simulink model "bee_scratch"  (Simulink 7.0)
settings: Solver=ode45  StartTime=0.0  StopTime=600  RelTol=1e-3
libraries: xbsIndex_r4 x52, xps_library x7, casper_library x2
settings Model: Creator=Laura  LastModifiedBy=Laura

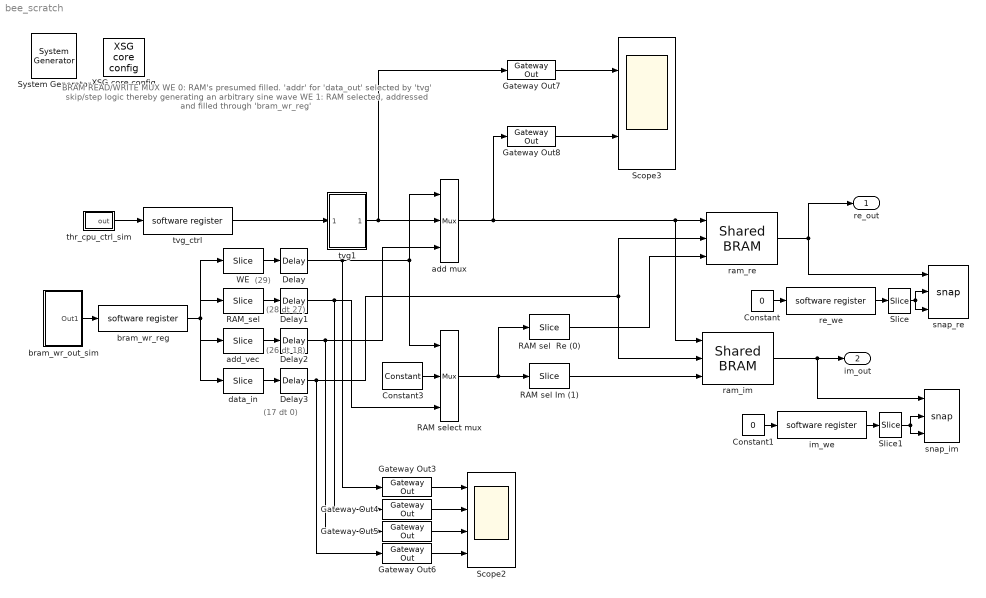
== system bee_scratch ==
  note: BRAM READ/WRITE MUX
      | WE 0: RAM's presumed filled.
      | 'addr' for 'data_out' selected
      | by 'tvg' skip/step logic thereby
      | generating an arbitrary sine wave
      | WE 1: RAM selected, addressed
      | and filled through
      | 'bram_wr_reg'
  note: (29)
  note: (28 dt 27)
  note: (17 dt 0)
  note: (26 dt 18)
  " System Generator" : xbsIndex_r4/ System Generator  Tag=genX  SystemSampleTime=-1  xilinxfamily=virtex2p  part=xc2vp70  speed=-7  package=ff1704  synthesis_tool=XST  clock_wrapper=Clock Enables  directory=./bee_scratch/sysgen  testbench=off  simulink_period=1  sysclk_period=5  dcm_input_clock_period=100  incr_netlist=off  trim_vbits=Everywhere in SubSystem  dbl_ovrd=According to Block Masks  core_generation=According to Block Masks  run_coregen=off  deprecated_control=off  eval_field=0  block_type=sysgen
      settings: block_version=10.1.2
  Constant : Constant  Value=0  OutDataType=sfix(16)  OutScaling=2^0
  Constant1 : Constant  Value=0  OutDataType=sfix(16)  OutScaling=2^0
  Constant3 : xbsIndex_r4/Constant  arith_type=Unsigned  const=0  n_bits=4  bin_pt=0  explicit_period=on  period=1  equ=P=C  opselect=C  inp2=PCIN>>17  opr=+  inp1=P  carry=CIN  dbl_ovrd=off  block_type=constant
      settings: block_version=10.1.2
  Delay{,1..3} (4 alike) : xbsIndex_r4/Delay  en=off  latency=1  dbl_ovrd=off  reg_retiming=off  block_type=delay
      settings: xl_area=[0, 0, 0, 0, 0, 0, 0]  block_version=10.1.2
  Gateway Out{3..8} (6 alike) : xbsIndex_r4/Gateway Out  hdl_port=on  timing_constraint=None  locs_specified=off  LOCs={}  block_type=gatewayout
      settings: infoedit="Gateway out block.  Converts Xilinx fixed point inputs into ouputs of type Simulink integer, double, or fixed point.<P><P>Hardware notes:  In hardware these blocks become top level output ports or are discarded, depending on how they are configured."  xl_area=[0, 0, 0, 0, 0, 0, 0]  block_version=10.1.2
  RAM sel  Re (0) : xbsIndex_r4/Slice  nbits=1  boolean_output=on  mode=Lower Bit Location + Width  bit1=0  base1=MSB of Input  bit0=0  base0=LSB of Input  dbl_ovrd=off  block_type=slice
      settings: infoedit="Extracts a given range of bits from each input sample and presents it at the output.  The output type is ordinarily unsigned with binary point at zero, but can be Boolean when the slice is one bit wide.<P><P>Hardware notes: In hardware this block costs nothing."  block_version=10.1.2
  RAM sel Im (1) : xbsIndex_r4/Slice  nbits=1  boolean_output=on  mode=Lower Bit Location + Width  bit1=0  base1=MSB of Input  bit0=1  base0=LSB of Input  dbl_ovrd=off  block_type=slice
      settings: infoedit="Extracts a given range of bits from each input sample and presents it at the output.  The output type is ordinarily unsigned with binary point at zero, but can be Boolean when the slice is one bit wide.<P><P>Hardware notes: In hardware this block costs nothing."  block_version=10.1.2
  RAM select mux : xbsIndex_r4/Mux  inputs=2  en=off  latency=0  precision=Full  arith_type="Signed  (2's comp)"  n_bits=8  bin_pt=2  quantization=Truncate  overflow=Wrap  dbl_ovrd=off  block_type=mux
      settings: xl_area=[0, 0, 0, 0, 0, 0, 0]  block_version=10.1.2
  RAM_sel : xbsIndex_r4/Slice  nbits=2  boolean_output=off  mode=Lower Bit Location + Width  bit1=10  base1=MSB of Input  bit0=27  base0=LSB of Input  dbl_ovrd=off  block_type=slice
      settings: infoedit="Extracts a given range of bits from each input sample and presents it at the output.  The output type is ordinarily unsigned with binary point at zero, but can be Boolean when the slice is one bit wide.<P><P>Hardware notes: In hardware this block costs nothing."  block_version=10.1.2
  Scope2 : Scope  NumInputPorts=4
      settings: YMin=-5~-5~-5~-5  YMax=5~5~5~5
  Scope3 : Scope  NumInputPorts=2
      settings: YMin=-5~-5  YMax=5~5  SaveName=ScopeData3
  Slice : xbsIndex_r4/Slice  nbits=1  boolean_output=on  mode=Lower Bit Location + Width  bit1=0  base1=MSB of Input  bit0=0  base0=LSB of Input  dbl_ovrd=off  block_type=slice
      settings: infoedit="Extracts a given range of bits from each input sample and presents it at the output.  The output type is ordinarily unsigned with binary point at zero, but can be Boolean when the slice is one bit wide.<P><P>Hardware notes: In hardware this block costs nothing."  block_version=10.1.2
  Slice1 : xbsIndex_r4/Slice  nbits=1  boolean_output=on  mode=Lower Bit Location + Width  bit1=0  base1=MSB of Input  bit0=0  base0=LSB of Input  dbl_ovrd=off  block_type=slice
      settings: infoedit="Extracts a given range of bits from each input sample and presents it at the output.  The output type is ordinarily unsigned with binary point at zero, but can be Boolean when the slice is one bit wide.<P><P>Hardware notes: In hardware this block costs nothing."  block_version=10.1.2
  WE : xbsIndex_r4/Slice  nbits=1  boolean_output=off  mode=Lower Bit Location + Width  bit1=10  base1=MSB of Input  bit0=29  base0=LSB of Input  dbl_ovrd=off  block_type=slice
      settings: infoedit="Extracts a given range of bits from each input sample and presents it at the output.  The output type is ordinarily unsigned with binary point at zero, but can be Boolean when the slice is one bit wide.<P><P>Hardware notes: In hardware this block costs nothing."  block_version=10.1.2
  XSG core config : xps_library/XSG core config  Tag=xps:xsg  SystemSampleTime=-1  hw_sys=BEE2_usr  ibob_linux=off  clk_src=usr_clk2x  gpio_clk_io_group=iBOB:sma  gpio_clk_bit_index=0  clk_rate=200  sample_period=1  synthesis_tool=XST  mpc_type=powerpc405
  add mux : xbsIndex_r4/Mux  inputs=2  en=off  latency=0  precision=Full  arith_type="Signed  (2's comp)"  n_bits=8  bin_pt=2  quantization=Truncate  overflow=Wrap  dbl_ovrd=off  block_type=mux
      settings: xl_area=[0, 0, 0, 0, 0, 0, 0]  block_version=10.1.2
  add_vec : xbsIndex_r4/Slice  nbits=9  boolean_output=off  mode=Lower Bit Location + Width  bit1=0  base1=MSB of Input  bit0=18  base0=LSB of Input  dbl_ovrd=off  block_type=slice
      settings: infoedit="Extracts a given range of bits from each input sample and presents it at the output.  The output type is ordinarily unsigned with binary point at zero, but can be Boolean when the slice is one bit wide.<P><P>Hardware notes: In hardware this block costs nothing."  block_version=10.1.2
  bram_wr_out_sim : Subsystem  mask{we_enable=0, ram_sel=3, add_vec=512, data_in=32}
      mask prompts: we_enable "Write enable"; ram_sel "RAM selector (1 = Re; 2 = Im; 3 = both)"; add_vec "RAM address"; data_in "Data in"
  bram_wr_reg : xps_library/software register  Tag=xps:sw_reg  SystemSampleTime=-1  io_dir=From Processor  arith_type=Unsigned  bitwidth=32  bin_pt=0  sample_period=1  gw_name=bee_scratch_bram_wr_reg_user_data_out
      link override bee_scratch_bram_wr_reg_user_data_out: arith_type=Unsigned  n_bits=32  bin_pt=0  period=1
      link override bee_scratch_data_in_mux_tvg_in_bram_wr_reg_user_data_out: arith_type=Unsigned  n_bits=32  bin_pt=0  period=1
      link override bee_scratch_tvg_bram_wr_reg_user_data_out: arith_type=Unsigned  n_bits=32  bin_pt=0  period=1
      link override bee_scratch_tvg_in_bram_wr_reg_user_data_out: arith_type=Unsigned  n_bits=32  bin_pt=0  period=1
      link override testblk_uu_data_in_mux_tvg_in_bram_wr_reg_user_data_out: arith_type=Unsigned  n_bits=32  bin_pt=0  period=1
  data_in : xbsIndex_r4/Slice  nbits=18  boolean_output=off  mode=Lower Bit Location + Width  bit1=0  base1=MSB of Input  bit0=0  base0=LSB of Input  dbl_ovrd=off  block_type=slice
      settings: infoedit="Extracts a given range of bits from each input sample and presents it at the output.  The output type is ordinarily unsigned with binary point at zero, but can be Boolean when the slice is one bit wide.<P><P>Hardware notes: In hardware this block costs nothing."  block_version=10.1.2
  im_we : xps_library/software register  Tag=xps:sw_reg  SystemSampleTime=-1  io_dir=From Processor  arith_type=Unsigned  bitwidth=32  bin_pt=0  sample_period=1  gw_name=bee_scratch_im_we_user_data_out
      link override bee_scratch_data_in_mux_tvg_in_im_we_user_data_out: arith_type=Unsigned  n_bits=32  bin_pt=0  period=1
      link override bee_scratch_im_we_user_data_out: arith_type=Unsigned  n_bits=32  bin_pt=0  period=1
      link override bee_scratch_tvg_im_we_user_data_out: arith_type=Unsigned  n_bits=32  bin_pt=0  period=1
      link override bee_scratch_tvg_in_im_we_user_data_out: arith_type=Unsigned  n_bits=32  bin_pt=0  period=1
      link override testblk_uu_data_in_mux_tvg_in_im_we_user_data_out: arith_type=Unsigned  n_bits=32  bin_pt=0  period=1
  ram_im : xps_library/Shared BRAM  Tag=xps:bram  SystemSampleTime=-1  arith_type="Signed  (2's comp)"  addr_width=11  data_width=32  data_bin_pt=0  init_vals=[1:2^11]  sample_rate=1
      link override bee_scratch_data_in_mux_tvg_in_ram_im_data_out: arith_type="Signed  (2's comp)"
      link override bee_scratch_ram_im_data_out: arith_type="Signed  (2's comp)"
      link override bee_scratch_tvg_in_ram_im_data_out: arith_type="Signed  (2's comp)"
      link override bee_scratch_tvg_ram_im_data_out: arith_type="Signed  (2's comp)"
      link override convert_din: arith_type="Signed  (2's comp)"
      link override mem/sim_data_in: arith_type="Signed  (2's comp)"
      link override testblk_uu_data_in_mux_tvg_in_ram_im_data_out: arith_type="Signed  (2's comp)"
  ram_re : xps_library/Shared BRAM  Tag=xps:bram  SystemSampleTime=-1  arith_type="Signed  (2's comp)"  addr_width=11  data_width=32  data_bin_pt=0  init_vals=[1:2^11]  sample_rate=1
      link override bee_scratch_data_in_mux_tvg_in_ram_re_data_out: arith_type="Signed  (2's comp)"
      link override bee_scratch_ram_re_data_out: arith_type="Signed  (2's comp)"
      link override bee_scratch_tvg_in_ram_re_data_out: arith_type="Signed  (2's comp)"
      link override bee_scratch_tvg_ram_re_data_out: arith_type="Signed  (2's comp)"
      link override convert_din: arith_type="Signed  (2's comp)"
      link override mem/sim_data_in: arith_type="Signed  (2's comp)"
      link override testblk_uu_data_in_mux_tvg_in_ram_re_data_out: arith_type="Signed  (2's comp)"
  re_we : xps_library/software register  Tag=xps:sw_reg  SystemSampleTime=-1  io_dir=From Processor  arith_type=Unsigned  bitwidth=32  bin_pt=0  sample_period=1  gw_name=bee_scratch_re_we_user_data_out
      link override bee_scratch_data_in_mux_tvg_in_re_we_user_data_out: arith_type=Unsigned  n_bits=32  bin_pt=0  period=1
      link override bee_scratch_re_we_user_data_out: arith_type=Unsigned  n_bits=32  bin_pt=0  period=1
      link override bee_scratch_tvg_in_re_we_user_data_out: arith_type=Unsigned  n_bits=32  bin_pt=0  period=1
      link override bee_scratch_tvg_re_we_user_data_out: arith_type=Unsigned  n_bits=32  bin_pt=0  period=1
      link override testblk_uu_data_in_mux_tvg_in_re_we_user_data_out: arith_type=Unsigned  n_bits=32  bin_pt=0  period=1
  snap_im : casper_library/Scopes/snap  SystemSampleTime=-1  nsamples=11
      link override addr/convert: arith_type=Unsigned  n_bits=32  bin_pt=0
      link override bram/bee_scratch_data_in_mux_tvg_in_snap_im_bram_data_out: arith_type=Unsigned
      link override bram/bee_scratch_snap_im_bram_data_out: arith_type=Unsigned
      link override bram/bee_scratch_tvg_in_snap_im_bram_data_out: arith_type=Unsigned
      link override bram/bee_scratch_tvg_snap_im_bram_data_out: arith_type=Unsigned
      link override bram/convert_din: arith_type=Unsigned
      link override bram/mem/sim_data_in: arith_type=Unsigned
      link override bram/testblk_uu_data_in_mux_tvg_in_snap_im_bram_data_out: arith_type=Unsigned
      link override ctrl/bee_scratch_data_in_mux_tvg_in_snap_im_ctrl_user_data_out: arith_type=Unsigned  n_bits=32  bin_pt=0  period=1
      link override ctrl/bee_scratch_snap_im_ctrl_user_data_out: arith_type=Unsigned  n_bits=32  bin_pt=0  period=1
      link override ctrl/bee_scratch_tvg_in_snap_im_ctrl_user_data_out: arith_type=Unsigned  n_bits=32  bin_pt=0  period=1
      link override ctrl/bee_scratch_tvg_snap_im_ctrl_user_data_out: arith_type=Unsigned  n_bits=32  bin_pt=0  period=1
      link override ctrl/testblk_uu_data_in_mux_tvg_in_snap_im_ctrl_user_data_out: arith_type=Unsigned  n_bits=32  bin_pt=0  period=1
  snap_re : casper_library/Scopes/snap  SystemSampleTime=-1  nsamples=11
      link override addr/convert: arith_type=Unsigned  n_bits=32  bin_pt=0
      link override bram/bee_scratch_data_in_mux_tvg_in_snap_re_bram_data_out: arith_type=Unsigned
      link override bram/bee_scratch_snap_re_bram_data_out: arith_type=Unsigned
      link override bram/bee_scratch_tvg_in_snap_re_bram_data_out: arith_type=Unsigned
      link override bram/bee_scratch_tvg_snap_re_bram_data_out: arith_type=Unsigned
      link override bram/convert_din: arith_type=Unsigned
      link override bram/mem/sim_data_in: arith_type=Unsigned
      link override bram/testblk_uu_data_in_mux_tvg_in_snap_re_bram_data_out: arith_type=Unsigned
      link override ctrl/bee_scratch_data_in_mux_tvg_in_snap_re_ctrl_user_data_out: arith_type=Unsigned  n_bits=32  bin_pt=0  period=1
      link override ctrl/bee_scratch_snap_re_ctrl_user_data_out: arith_type=Unsigned  n_bits=32  bin_pt=0  period=1
      link override ctrl/bee_scratch_tvg_in_snap_re_ctrl_user_data_out: arith_type=Unsigned  n_bits=32  bin_pt=0  period=1
      link override ctrl/bee_scratch_tvg_snap_re_ctrl_user_data_out: arith_type=Unsigned  n_bits=32  bin_pt=0  period=1
      link override ctrl/testblk_uu_data_in_mux_tvg_in_snap_re_ctrl_user_data_out: arith_type=Unsigned  n_bits=32  bin_pt=0  period=1
  thr_cpu_ctrl_sim : Subsystem  mask{tvg_skip=3, tvg_stall=2, tvg_length=145}
      mask prompts: tvg_skip "Skip"; tvg_stall "Stall"; tvg_length "Length"
      mask help:
      | Mux Data for CT and FFT Syncs:
      |
      | 0 -> Interchip Connection
      | 1 -> User Generated External Sync
      | 2 -> Periodic Sync Generator
      | 3 -> Periodic Sync Generator (Same as 2)
      |
      | Mux Data for CT and FFT Inputs:
      |
      | 0 -> Interchip Connection
      | 1 -> Test Vector Generator (TVG)
      | 2 -> All Zeroes (0's)
      | 3 -> All Ones (1's)
  tvg1 : Subsystem  mask(Test Vector Generator(TVG)){tvg_skip=1, tvg_stall=1, tvg_length=512}
      mask prompts: tvg_skip "Skip"; tvg_stall "Stall"; tvg_length "Length"
  tvg_ctrl : xps_library/software register  Tag=xps:sw_reg  SystemSampleTime=-1  io_dir=From Processor  arith_type=Unsigned  bitwidth=32  bin_pt=0  sample_period=1  gw_name=bee_scratch_tvg_ctrl_user_data_out
      link override bee_scratch_data_in_mux_tvg_in_tvg_ctrl_user_data_out: arith_type=Unsigned  n_bits=32  bin_pt=0  period=1
      link override bee_scratch_tvg_ctrl_user_data_out: arith_type=Unsigned  n_bits=32  bin_pt=0  period=1
      link override bee_scratch_tvg_in_tvg_ctrl_user_data_out: arith_type=Unsigned  n_bits=32  bin_pt=0  period=1
      link override bee_scratch_tvg_tvg_ctrl_user_data_out: arith_type=Unsigned  n_bits=32  bin_pt=0  period=1
      link override testblk_uu_data_in_mux_tvg_in_tvg_ctrl_user_data_out: arith_type=Unsigned  n_bits=32  bin_pt=0  period=1
  re_out : Outport  OutDataType=sfix(16)  OutScaling=2^0
  im_out : Outport  Port=2  OutDataType=sfix(16)  OutScaling=2^0
  wires:
  ram_im/1 -> im_out/1, snap_im/1
  ram_re/1 -> re_out/1, snap_re/1
  bram_wr_out_sim/1(Out1) -> bram_wr_reg/1
  thr_cpu_ctrl_sim/1(out) -> tvg_ctrl/1
  tvg_ctrl/1 -> tvg1/1(In1)
  tvg1/1(Out1) -> Gateway Out7/1, add mux/2
  Constant3/1 -> RAM select mux/2
  RAM select mux/1 -> RAM sel Im (1)/1, RAM sel  Re (0)/1
  RAM sel  Re (0)/1 -> ram_re/3
  WE/1 -> Delay/1
  bram_wr_reg/1 -> WE/1, RAM_sel/1, add_vec/1, data_in/1
  add_vec/1 -> Delay2/1
  RAM_sel/1 -> Delay1/1
  add mux/1 -> Gateway Out8/1, ram_re/1, ram_im/1
  data_in/1 -> Delay3/1
  RAM sel Im (1)/1 -> ram_im/3
  Gateway Out3/1 -> Scope2/1
  Gateway Out4/1 -> Scope2/2
  Gateway Out5/1 -> Scope2/3
  Gateway Out6/1 -> Scope2/4
  Delay/1 -> RAM select mux/1, add mux/1, Gateway Out3/1
  Delay1/1 -> RAM select mux/3, Gateway Out4/1
  Delay2/1 -> add mux/3, Gateway Out5/1
  Delay3/1 -> ram_re/2, ram_im/2, Gateway Out6/1
  Gateway Out7/1 -> Scope3/1
  Gateway Out8/1 -> Scope3/2
  Slice/1 -> snap_re/3, snap_re/2
  re_we/1 -> Slice/1
  Constant/1 -> re_we/1
  Slice1/1 -> snap_im/3, snap_im/2
  im_we/1 -> Slice1/1
  Constant1/1 -> im_we/1

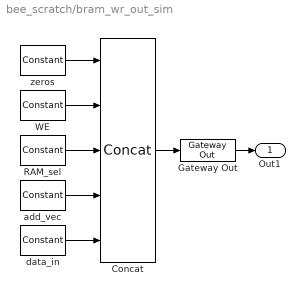
== system bee_scratch/bram_wr_out_sim ==
  Concat : xbsIndex_r4/Concat  num_inputs=5  dbl_ovrd=off  block_type=concat
      settings: block_version=10.1.2
  Gateway Out : xbsIndex_r4/Gateway Out  hdl_port=on  timing_constraint=None  locs_specified=off  LOCs={}  block_type=gatewayout
      settings: infoedit="Gateway out block.  Converts Xilinx fixed point inputs into ouputs of type Simulink integer, double, or fixed point.<P><P>Hardware notes:  In hardware these blocks become top level output ports or are discarded, depending on how they are configured."  xl_area=[0, 0, 0, 0, 0, 0, 0]  block_version=10.1.2
  RAM_sel : xbsIndex_r4/Constant  arith_type=Unsigned  const=ram_sel  n_bits=2  bin_pt=0  explicit_period=on  period=1  equ=P=C  opselect=C  inp2=PCIN>>17  opr=+  inp1=P  carry=CIN  dbl_ovrd=off  block_type=constant
      settings: block_version=10.1.2
  WE : xbsIndex_r4/Constant  arith_type=Unsigned  const=we_enable  n_bits=1  bin_pt=0  explicit_period=on  period=1  equ=P=C  opselect=C  inp2=PCIN>>17  opr=+  inp1=P  carry=CIN  dbl_ovrd=off  block_type=constant
      settings: block_version=10.1.2
  add_vec : xbsIndex_r4/Constant  arith_type=Unsigned  const=add_vec  n_bits=9  bin_pt=0  explicit_period=on  period=1  equ=P=C  opselect=C  inp2=PCIN>>17  opr=+  inp1=P  carry=CIN  dbl_ovrd=off  block_type=constant
      settings: block_version=10.1.2
  data_in : xbsIndex_r4/Constant  arith_type=Unsigned  const=data_in  n_bits=18  bin_pt=0  explicit_period=on  period=1  equ=P=C  opselect=C  inp2=PCIN>>17  opr=+  inp1=P  carry=CIN  dbl_ovrd=off  block_type=constant
      settings: block_version=10.1.2
  zeros : xbsIndex_r4/Constant  arith_type=Unsigned  const=0  n_bits=2  bin_pt=0  explicit_period=on  period=1  equ=P=C  opselect=C  inp2=PCIN>>17  opr=+  inp1=P  carry=CIN  dbl_ovrd=off  block_type=constant
      settings: block_version=10.1.2
  Out1 : Outport  OutDataType=sfix(16)  OutScaling=2^0
  wires:
  Gateway Out/1 -> Out1/1
  Concat/1 -> Gateway Out/1
  zeros/1 -> Concat/1
  WE/1 -> Concat/2
  RAM_sel/1 -> Concat/3
  add_vec/1 -> Concat/4
  data_in/1 -> Concat/5

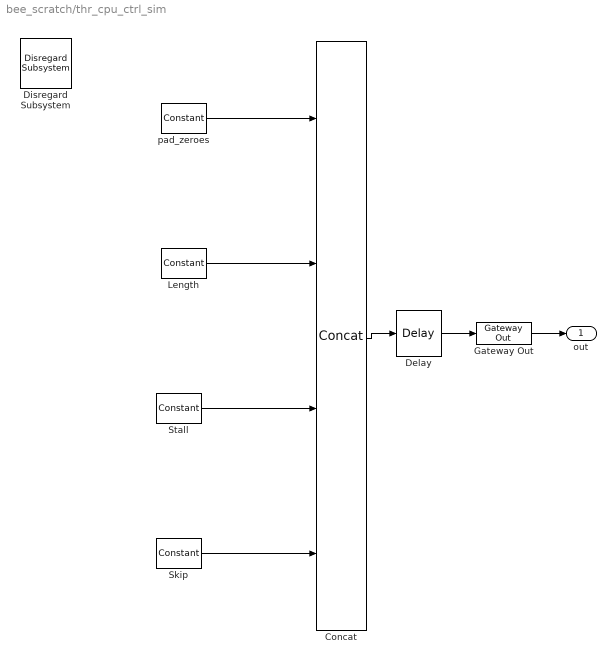
== system bee_scratch/thr_cpu_ctrl_sim ==
  Concat : xbsIndex_r4/Concat  num_inputs=4  dbl_ovrd=off  block_type=concat
      settings: block_version=10.1.2
  Delay : xbsIndex_r4/Delay  en=off  latency=1  dbl_ovrd=off  reg_retiming=off  block_type=delay
      settings: xl_area=[0, 0, 0, 0, 0, 0, 0]  block_version=10.1.2
  Disregard Subsystem : xbsIndex_r4/Disregard Subsystem  Tag=discardX  block_type=disregard
      settings: block_version=10.1.2
  Gateway Out : xbsIndex_r4/Gateway Out  hdl_port=off  timing_constraint=None  locs_specified=off  LOCs={}  block_type=gatewayout
      settings: infoedit="Gateway out block.  Converts Xilinx fixed point inputs into ouputs of type Simulink integer, double, or fixed point.<P><P>Hardware notes:  In hardware these blocks become top level output ports or are discarded, depending on how they are configured."  xl_area=[0, 0, 0, 0, 0, 0, 0]  block_version=10.1.2
  Length : xbsIndex_r4/Constant  arith_type=Unsigned  const=tvg_length  n_bits=10  bin_pt=0  explicit_period=on  period=1  equ=P=C  opselect=C  inp2=PCIN>>17  opr=+  inp1=P  carry=CIN  dbl_ovrd=off  block_type=constant
      settings: block_version=10.1.2
  "Skip\t" : xbsIndex_r4/Constant  arith_type=Unsigned  const=tvg_skip  n_bits=10  bin_pt=0  explicit_period=on  period=1  equ=P=C  opselect=C  inp2=PCIN>>17  opr=+  inp1=P  carry=CIN  dbl_ovrd=off  block_type=constant
      settings: block_version=10.1.2
  Stall : xbsIndex_r4/Constant  arith_type=Unsigned  const=tvg_stall  n_bits=10  bin_pt=0  explicit_period=on  period=1  equ=P=C  opselect=C  inp2=PCIN>>17  opr=+  inp1=P  carry=CIN  dbl_ovrd=off  block_type=constant
      settings: block_version=10.1.2
  pad_zeroes : xbsIndex_r4/Constant  arith_type=Unsigned  const=0  n_bits=2  bin_pt=0  explicit_period=on  period=1  equ=P=C  opselect=C  inp2=PCIN>>17  opr=+  inp1=P  carry=CIN  dbl_ovrd=off  block_type=constant
      settings: block_version=10.1.2
  out : Outport  OutDataType=sfix(16)  OutScaling=2^0
  wires:
  "Skip\t"/1 -> Concat/4
  Delay/1 -> Gateway Out/1
  Concat/1 -> Delay/1
  Gateway Out/1 -> out/1
  Stall/1 -> Concat/3
  pad_zeroes/1 -> Concat/1
  Length/1 -> Concat/2

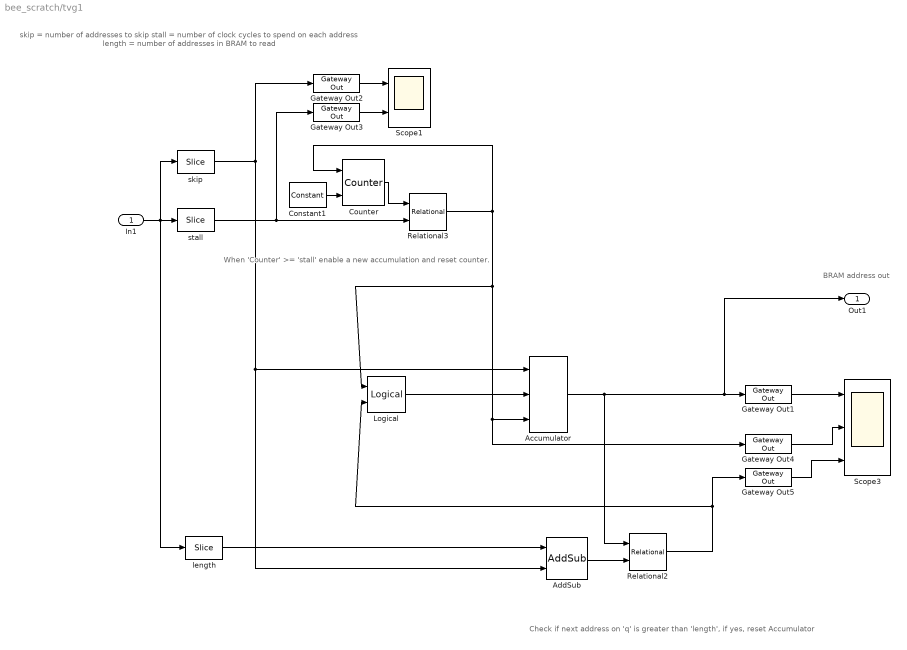
== system bee_scratch/tvg1 ==
  note: BRAM address out
  note: Check if next address on 'q'
      | is greater than 'length',
      | if yes, reset Accumulator
  note: When 'Counter' >= 'stall'
      | enable a new accumulation
      | and reset counter.
  note: skip = number of addresses to skip
      | stall = number of clock cycles to spend
      | on each address
      | length = number of addresses in BRAM
      | to read
  In1 : Inport  OutDataType=sfix(16)  OutScaling=2^0
  Accumulator : xbsIndex_r4/Accumulator  operation=Add  n_bits=10  overflow=Wrap  scale=1  rst=on  hasbypass=off  en=on  dbl_ovrd=off  use_behavioral_HDL=on  block_type=accum
      settings: infoedit="Adder or subtractor-based accumulator.   Output type and binary point position match the input.<P><P>Hardware notes: When \"Reinitialize with input 'b' on reset\" is selected, the accumulator is forced to run at the system rate even if the input 'b' is running at a slower rate."  xl_area=[0, 0, 0, 0, 0, 0, 0]  block_version=10.1.2
  AddSub : xbsIndex_r4/AddSub  mode=Subtraction  use_carryin=off  use_carryout=off  en=off  latency=1  precision=Full  arith_type=Unsigned  n_bits=8  bin_pt=2  quantization=Truncate  overflow=Wrap  dbl_ovrd=off  use_behavioral_HDL=on  pipelined=off  use_rpm=on  block_type=addsub
      settings: xl_area=[0, 0, 0, 0, 0, 0, 0]  block_version=10.1.2
  Constant1 : xbsIndex_r4/Constant  arith_type=Unsigned  const=1  n_bits=10  bin_pt=0  explicit_period=on  period=1  equ=P=C  opselect=C  inp2=PCIN>>17  opr=+  inp1=P  carry=CIN  dbl_ovrd=off  block_type=constant
      settings: block_version=10.1.2
  Counter : xbsIndex_r4/Counter  cnt_type=Free Running  cnt_to=inf  operation=Up  start_count=0  cnt_by_val=1  arith_type=Unsigned  n_bits=10  bin_pt=0  load_pin=on  rst=off  en=off  explicit_period=on  period=1  dbl_ovrd=off  use_behavioral_HDL=off  use_rpm=on  block_type=counter
      settings: xl_area=[0, 0, 0, 0, 0, 0, 0]  block_version=10.1.2
  Gateway Out{1..5} (5 alike) : xbsIndex_r4/Gateway Out  hdl_port=on  timing_constraint=None  locs_specified=off  LOCs={}  block_type=gatewayout
      settings: infoedit="Gateway out block.  Converts Xilinx fixed point inputs into ouputs of type Simulink integer, double, or fixed point.<P><P>Hardware notes:  In hardware these blocks become top level output ports or are discarded, depending on how they are configured."  xl_area=[0, 0, 0, 0, 0, 0, 0]  block_version=10.1.2
  Logical : xbsIndex_r4/Logical  logical_function=AND  inputs=2  en=off  latency=0  precision=Full  arith_type=Unsigned  n_bits=8  bin_pt=2  align_bp=on  dbl_ovrd=off  block_type=logical
      settings: xl_area=[0, 0, 0, 0, 0, 0, 0]  block_version=10.1.2
  Relational2 : xbsIndex_r4/Relational  mode=a>=b  en=off  latency=0  dbl_ovrd=off  block_type=relational
      settings: xl_area=[0, 0, 0, 0, 0, 0, 0]  block_version=10.1.2
  Relational3 : xbsIndex_r4/Relational  mode=a>=b  en=off  latency=0  dbl_ovrd=off  block_type=relational
      settings: xl_area=[0, 0, 0, 0, 0, 0, 0]  block_version=10.1.2
  Scope1 : Scope  NumInputPorts=2
      settings: YMin=-5~-5  YMax=5~5
  Scope3 : Scope  NumInputPorts=3
      settings: TimeRange=20  YMin=-5~-5~-5  YMax=5~5~5  SaveName=ScopeData4
  length : xbsIndex_r4/Slice  nbits=10  boolean_output=off  mode=Lower Bit Location + Width  bit1=0  base1=MSB of Input  bit0=20  base0=LSB of Input  dbl_ovrd=off  block_type=slice
      settings: infoedit="Extracts a given range of bits from each input sample and presents it at the output.  The output type is ordinarily unsigned with binary point at zero, but can be Boolean when the slice is one bit wide.<P><P>Hardware notes: In hardware this block costs nothing."  block_version=10.1.2
  skip : xbsIndex_r4/Slice  nbits=10  boolean_output=off  mode=Lower Bit Location + Width  bit1=0  base1=MSB of Input  bit0=0  base0=LSB of Input  dbl_ovrd=off  block_type=slice
      settings: infoedit="Extracts a given range of bits from each input sample and presents it at the output.  The output type is ordinarily unsigned with binary point at zero, but can be Boolean when the slice is one bit wide.<P><P>Hardware notes: In hardware this block costs nothing."  block_version=10.1.2
  stall : xbsIndex_r4/Slice  nbits=10  boolean_output=off  mode=Lower Bit Location + Width  bit1=0  base1=MSB of Input  bit0=10  base0=LSB of Input  dbl_ovrd=off  block_type=slice
      settings: infoedit="Extracts a given range of bits from each input sample and presents it at the output.  The output type is ordinarily unsigned with binary point at zero, but can be Boolean when the slice is one bit wide.<P><P>Hardware notes: In hardware this block costs nothing."  block_version=10.1.2
  Out1 : Outport  OutDataType=sfix(16)  OutScaling=2^0
  wires:
  In1/1 -> stall/1, skip/1, length/1
  Gateway Out1/1 -> Scope3/1
  skip/1 -> Gateway Out2/1, Accumulator/1, AddSub/2
  stall/1 -> Gateway Out3/1, Relational3/2
  Gateway Out2/1 -> Scope1/1
  Gateway Out3/1 -> Scope1/2
  Gateway Out4/1 -> Scope3/2
  Relational3/1 -> Counter/1, Accumulator/3, Gateway Out4/1, Logical/1
  Counter/1 -> Relational3/1
  Constant1/1 -> Counter/2
  Relational2/1 -> Logical/2, Gateway Out5/1
  Logical/1 -> Accumulator/2
  Accumulator/1 -> Relational2/1, Gateway Out1/1, Out1/1
  length/1 -> AddSub/1
  AddSub/1 -> Relational2/2
  Gateway Out5/1 -> Scope3/3
